simulink model "SCS"  (R2025a)
settings: Solver=ode45  StartTime=0.0  StopTime=1  RelTol=1e-3
settings Model: Creator=JR  LastModifiedBy=JR

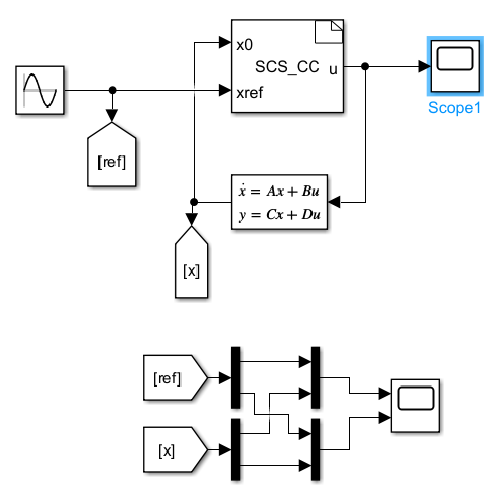
[thumbnail: Simulink's stored preview of the top-level diagram]
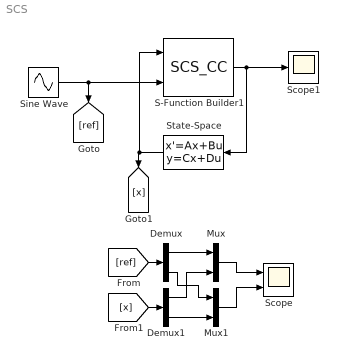
== system SCS ==
  Demux : Demux  Outputs=2
  Demux1 : Demux  Outputs=2
  Mux : Mux  Inputs=2
  Mux1 : Mux  Inputs=2
  S-Function Builder1 : S-Function  FunctionName=SCS_CC  SFunctionModules=SCS_CC_wrapper.c cpg_solve cpg_workspace aa cones ctrlc linalg normalize rw scs scs_version util scs_matrix csparse qdldl amd_1 amd_2 amd_aat amd_control amd_defaults amd_dump amd_global amd_info amd_order amd_post_tree amd_postorder amd_preprocess amd_valid SuiteSparse_config private  SFunctionDeploymentMode=off  EnableBusSupport=off  mask(S-Function Builder){}
      mask help: Simulink:masks:SFunctionBuilder_MD
      mask init:
      | val = [[.9  0.75 0.75 1 1 .9 .9 1]',[1 1 0.75 0.75 .9 .9 1 .9]'];try , sys = get_param(gcb,'SfunBuilderFcnName');if isempty(sys), sys = get_param(gcb,'FunctionName'); end,catch, sys = get_param(gcb,'FunctionName'); end
      settings: CopyFcn=set_param(gcbh,'LinkStatus','none')  OpenFcn=sfunctionwizard(gcbh)
      mask Display:
      | plot(val(:,1),val(:,2))
      | disp(sys)
      | port_label('input',1,sprintf('%s', 'x0'),'interpreter','tex')
      | port_label('input',2,sprintf('%s', 'xref'),'interpreter','tex')
      | port_label('output',1,sprintf('%s', 'u'),'interpreter','tex')
  Scope : Scope  NumInputPorts=2
      settings: ActiveDisplayYMinimum=-2.4999999680253175  ActiveDisplayYMaximum=2.4999999964472575
  Scope1 : Scope
      settings: ActiveDisplayYMinimum=-38.461537715485349  ActiveDisplayYMaximum=38.461537715485349
  Sine Wave : Sin  Amplitude=[1;1]  Frequency=100  Phase=[0;pi/2]  SampleTime=0
  State-Space : StateSpace  A=[0 0;0 0]  B=[-400 0; 0 -400]  C=[1 0;0 1]  D=[0 0;0 0]  InitialCondition=[2 ;-1]
  wires:
  S-Function Builder1/1 -> State-Space/1, Scope1/1
  Sine Wave/1 -> [ref], S-Function Builder1/2
  State-Space/1 -> [x], S-Function Builder1/1
  Demux1/1 -> Mux/2
  Demux/1 -> Mux/1
  Mux/1 -> Scope/1
  Demux/2 -> Mux1/1
  Demux1/2 -> Mux1/2
  Mux1/1 -> Scope/2
  [ref] -> Demux/1
  [x] -> Demux1/1
